simulink model "RB_KAIROS_BaseOnly"  (R2020b)
settings: Solver=ode4  StartTime=0.0  StopTime=t_end  FixedStep=Ts  RelTol=1e-3
values from neighbouring files (symbols this model uses):
  am = 0.3    [RB_KAIROS_ImpControl_OpSpace_BaseOnly.m]
  am_r = 0.3    [RB_KAIROS_ImpControl_OpSpace_BaseOnly.m]
  Jv = [1 0 0; 0 1 0; 0 0 0; 0 0 0; 0 0 0; 0 0 1;]    [RB_KAIROS_ImpControl_OpSpace_BaseOnly.m]
  Kc = diag(5*[1000,1000,0,0,0,1000])    [RB_KAIROS_ImpControl_OpSpace_BaseOnly.m]
  model_sample_time = 0.001    [RB_KAIROS_ImpControl_OpSpace_BaseOnly.m]
  q_dot_0 = zeros(10,1)    [RB_KAIROS_ImpControl_OpSpace_BaseOnly.m]
  T_i = T_W_V    [RB_KAIROS_ImpControl_OpSpace_BaseOnly.m]
  tau_ext = [0 0 0]    [RB_KAIROS_ImpControl_OpSpace_BaseOnly.m]
  v_SMU = 10    [RB_KAIROS_ImpControl_OpSpace_BaseOnly.m]
  vm = 0.6    [RB_KAIROS_ImpControl_OpSpace_BaseOnly.m]
  vm_r = 0.6    [RB_KAIROS_ImpControl_OpSpace_BaseOnly.m]
undefined symbols (not defined in the file or in its folder): DiscIntNeverNeededParam, magnitude, q_0, T_f
libraries: simulink x4, utils x4, transformations_lib x1
(part 14 of 16)

== matlab function RB_KAIROS_BaseOnly/CONTROLLER /Kinematics and Dynamics/Kinematics - error representation/MATLAB Function2 ==
  data: R_D_W_aug input; vt output; x_dot_d input; x_ddot_d input; vt_dot output; x_err input; x_dot_err input
function [vt, vt_dot] = compute_vt(R_D_W_aug, x_dot_d, x_ddot_d, x_err, x_dot_err)
% This function is used to compute the vectors vt and vt_dot defined in Ott book in order
% to convert the equation of motion to an equivalent representation using
% error on the task variables

% INPUTS:
% - R_W_D_aug is an extension of the ROTATION MATRIX from world frame to 
%   desired frame: [R_W_D 0; 0 R_W_D], it is a 6x6 matrix
% - omega_d, p_dot_d, p_err, eps_err, omega_err are all quantities defined in
%   the world frame (or space frame) W.
S_omega_d = calc_skewsymm(x_dot_d(4:6));
S_alfa_d = calc_skewsymm(x_ddot_d(4:6));

a = [x_dot_d(1:3) + S_omega_d*(x_err(1:3));
                x_dot_d(4:6)];

vt = R_D_W_aug*a;

vt_dot = R_D_W_aug*(-augment_matrix(S_omega_d)*a + [x_ddot_d(1:3) + S_alfa_d*x_err(1:3) + S_omega_d*x_dot_err(1:3);
                                                                  x_ddot_d(4:6)]);

end 


function S = calc_skewsymm(v)

S = [0 -v(3) v(2);
    v(3) 0 -v(1);
    -v(2) v(1) 0];
end

function M_aug = augment_matrix(M)

M_aug = [M, zeros(3,3);
             zeros(3,3), M];
end

== matlab function RB_KAIROS_BaseOnly/CONTROLLER /Kinematics and Dynamics/Kinematics - error representation/MATLAB Function3 ==
  data: R_D_W_aug input; J_x output; J_b input
function J_x   =compute_J_x(R_D_W_aug, J_b)
% This function is used to compute the matrix J_x defined in Ott book in order
% to convert the equation of motion to an equivalent representation using
% error on the task variables

% INPUTS:
% - R_W_D_aug is an extension of the ROTATION MATRIX from world frame to 
%   desired frame: [R_W_D 0; 0 R_W_D], it is a 6x6 matrix
% - J_b is the body Jacobian of the robot 

J_x = R_D_W_aug*J_b;

== matlab function RB_KAIROS_BaseOnly/CONTROLLER /Primary task - Controller/MATLAB Function ==
  data: Kc input; Dc output; Lambda input
function Dc = compute_damping(Kc,Lambda)
%  COMPUTE_DAMPING Computes damping matrix to enforce desired second order
%  system behaviour.
%
%   Dc = COMPUTE_DAMPING(Kc,Lambda) computes the damping depending on 
%        stiffness matrix Kc (which has to be constant for stability) and
%        inertia matrix Lambda (which is time varying since no inertia 
%        shaping is applied).
%   
%   Reference: Cartesian Impedance Control of Redundant and Flexible-Joint
%              Robots, C. Ott 2005, page 36-37.
%   See also EIG

zeta = 1;

Lambda_3 = Lambda([1:2,6],[1:2,6]);
Kc_3 = Kc([1:2,6],[1:2,6])

A = real(sqrtm(Lambda_3));
Kc_1 = real(sqrtm(Kc_3));

D0 = zeta*eye(3,3);

Dc_3 = A*D0*Kc_1 + Kc_1*D0*A;

Dc = zeros(6,6);

Dc([1:2,6],[1:2,6]) = Dc_3

% DAMPING MATRIX (varying)
%Generalized eigenvalue decomposition for the pair (Kc,Lambda)
% Lambda_3 = Lambda([1:2,6],[1:2,6]);
% Kc_3 = Kc([1:2,6],[1:2,6]);
% [eigvecs,eigvals] =  eig(Kc_3, Lambda_3);
% eigvals = real(eigvals);
% eigvecs = real(eigvecs);
% %sorting eigs by magnitude
% % [eigvals,sidx] = sort(diag(eigvals),'descend');
% 
% %Finding matrices that satisfy K = Q'K0Q and Lambda = Q'*Q
% K0_3 = sqrt(eigvals);
% % V = eigvecs(:,sidx);
% Q_T = Lambda_3*eigvecs;
% Q = Q_T';
% 
% %Damping matrix computation
% zeta = 1*ones(3,1); %Imposing an overdamped behaviour
% D0_3 = diag(zeta).*K0_3;
% Dc_3 = 2*Q_T*D0_3*Q;
% 
% Dc = eye(6);
% Dc([1:2,6],[1:2,6]) = Dc_3

%OLD implementation where stiffness and damping were retrieven from
%configuration parameters
% function [Kc,Dc] = compute_stiffness_damping(J_T, J_i, J_d)
% 
% Kq_veh = [2850*ones(2,1); 750]; 
% Dq_veh = [2000;2000;800];
% 
% Kq = diag([Kq_veh]);
% Dq = diag([Dq_veh]);
% 
% Dc = J_i'*Dq*J_i;
% Kc = J_i'*(Kq-J_T*Dc*J_d)*J_i;
% end

== matlab function RB_KAIROS_BaseOnly/EE to task space quaternion quantities/Augment matrix ==
  data: R_W_D input; R_D_W_aug output
function R_D_W_aug = augment_matrix(R_W_D)

R_D_W_aug = [R_W_D', zeros(3,3);
             zeros(3,3), R_W_D'];

== matlab function RB_KAIROS_BaseOnly/Trajectory Generator/move2pose/Cartesian_ipol2/rotation/Embedded MATLAB Function1 ==
  data: t input; qd output; s0 input; v0 input; sf input; vm input; am input; dqd output; ddqd output; ipol_finished output; T_scale input; interpoly input
function [qd,dqd,ddqd, ipol_finished] = calc_qd(t,s0,v0,sf,vm,am,T_scale,interpoly)
% This function calculates a one dimensional movement with a trapezodial 
% signal for velocity over time. Additionally it is able to adapt to shifts
% in the maximum allowed velocity.
%
% Inputs:
% t         current runtime
% s0        start value for motion in position
% v0        start value for motion in velocity
% sf        final value for motion in position
% vm        maximum allowed velocity
% am        maximum allowed acceleration
% T_scale   Scaling factor for duration of adaption
% interpoly Which interpolation to use
%
% Outputs:
% qd        disered position at current time
% dqd       disered velocity at current time
% ddqd      disered acceleration at current time
% ipol_finished 
%           motion is finished

%% Initialize persistent variables for adaption motion
persistent vm1 adpt ti qi qf T t_shift
if isempty(vm1)
    vm1 = vm;       %remembers the max velocity from last run
end
if isempty(adpt)
    adpt = false;   %stores if an adaption motion is activated
end
if isempty(ti)
    ti = 0;         %Initial time step for adaption motion
end
if isempty(qi)
    qi = zeros(3,1);%Initial values (pos,vel,acc) for adaption motion
end
if isempty(qf)
    qf = zeros(3,1);%Final values (pos,vel,acc) for adaption motion
end
if isempty(T)
    T = 0;          %Duration of adaption motion; tf = ti+T
end
if isempty(t_shift)
    t_shift = 0;    %Time distance with which the current reference motion is shifted
end

% needed to delay tanhlog with one timestep
tanhlog_delay = 0;

%% This If runs only for one timestep!!!
% If current max velocity is unequal to old one 
% Not directly at the beginning
% Dont start new while a adaption is still running, to prevent reset of
%   initial values
if abs(vm-vm1)>1e-3 && t>0.001 && adpt==false                       
    adpt = true;          % Activate adaption
    ti = t;               % Set initial timestep to current step
    tanhlog_delay = 1;    % Activate the delay for tanhlog

    %%% inital set of position, velo, acceleration for adaption motion 
    % is the same as the old mogen would do (t_shift is not updated at
    % this time!)
    [qi, ~] = interpolator(ti+t_shift, compute_traj_parameters(s0, v0, sf, vm1, am));

    %%% computes the time shift for shifting the new motion to the end
    % point of the old motion. So at which time the new motion has
    % the same qd? Then calculate the time distance to the inital
    % time of the change in velocities
    % t_shift < 0 if new motion is faster (vm>vm1)
    % t_shift > 0 if new motion is slower (vm<vm1)
    % interpolator_1 is the inverse function of interpolator!
    t_shift = interpolator_1(qi(1), compute_traj_parameters(s0, v0, sf, vm, am)) - ti ;

    %%% Additional shift for adaption motion = Duration of adaption motion
    T_standard = abs(vm1-vm)/am;
    switch interpoly
        case 0
            T = 0;
            adpt = false;       %no adatption  
        case 1
            T = T_standard*2.2;    %tanhlog
        case 2
            T = (pi*abs(vm1-vm))/(2*am);  %Cosine version
        case 3
            T = T_standard;        %poly3
        case 4
            T = 1.5*(abs(vm1-vm)/am); %poly4
        case 5
            T = T_standard*1.5;        %poly5 
        case 7
            T = T_standard*1.75;        %poly7 
        otherwise
            T = T_standard;        %rest
    end

    % Scale Duration if needed
    T = T*T_scale;

    %%% The additional shift for adaption motion is dependent on the
    % difference in the velocities. See report for details.
    t_shift  = t_shift+(T/2)*((vm1/vm)-1);

    %%% Calculate final values for adaption motion. Which are reached
    % at inital time plus duration of adaption and new time shift
    [qf, ~] = interpolator(ti+t_shift+T, compute_traj_parameters(s0, v0, sf, vm, am));

end

%% Here the actual motion is calculated
% Interpolates the values of pos,vel,acc (qv) with parameters and current time t    
[qdv, ipol_finished] = interpolator(t+t_shift, compute_traj_parameters(s0, v0, sf, vm, am));  

%% If adaption motion needed
if adpt == true 

    %%% calculate the adaption moition, which takes time from ti to
    % ti+T. t is the current runtime, _i initial values, _f final
    % values, _m maximum values

    switch interpoly
        case 0
            adpt=false;                             %no adatption  
        case 1
            if tanhlog_delay == 1
                qdv = qi;  
                tanhlog_delay = 0;
            else
                qdv = tanhlog(t,ti,T,qi,qf,vm,am);      %tanhlog
            end
        case 2
            qdv = cosine(t,ti,T,qi,qf,vm,am);       %Cosine version
        case 3
            qdv = poly3(t,ti,T,qi,qf,vm,am);        %poly3
        case 4
            qdv = poly4(t,ti,T,qi,qf,vm,am);        %poly4
        case 5
            qdv = poly5(t,ti,T,qi,qf,vm,am);        %poly5 
        case 6
            qdv = poly6(t,ti,T,qi,qf,vm,am);        %poly6 
        case 7
            qdv = poly7(t,ti,T,qi,qf,vm,am);        %poly7 
        case 8
            qdv = poly4_mean(t,ti,T,qi,qf,vm,am);   %poly4_mean 
        case 9
            qdv = poly5_2mean(t,ti,T,qi,qf,vm,am);  %poly5_2mean 
        case 10
            qdv = tanhmean(t,ti,T,qi,qf,vm,am);     %tanhmean 
        otherwise
            error('Unknown adaption motion');       %rest
    end

    % If time is equal than the finish time => adaption motion is complete
    % But it is aborted one timestep earlier, since the finish timestep
    % is already computed correctly by the standard interpolator.
    if t >= (ti+T-0.001)
        adpt = false;     % If adaption finished => reset
    end
end

%% Set output
if sf == s0          % No motion needed if start = end 
    qd = s0;         % => set initial values
    dqd = v0;
    ddqd = 0;  
else     
    qd = qdv(1);     % set output
    dqd = qdv(2);
    ddqd = qdv(3);        
end

vm1 = vm;  %remember current max velocity

end

function [qv] = poly3(t,ti,T,qvi,qvf,dqm,ddqm)
%POLY3 computes a polynomial trajectory of degree 3 between initial (_i) 
%values and final (_f) values of position q, velocity dq and accelerataion
%ddq. Taken from Melchiorri presentation page 19

qi = qvi(1);      %split input vectors in pos,vel,acc
dqi = qvi(2);
ddqi = qvi(3);
qf = qvf(1);
dqf = qvf(2);
ddqf = qvf(3);
      
% current duration of motion dt
dt = t-ti;                      

% compute coefficients
a0 = qi;
a1 = dqi;
a2 = (-3*(qi-qf)-(2*dqi+dqf)*T)/(T^2);
a3 = (2*(qi-qf)+(dqi+dqf)*T)/(T^3);

% compute pos,vel,acc desired (_d)
qd = a0+a1*dt+a2*dt^2+a3*dt^3;
dqd = a1+2*a2*dt+3*a3*dt^2;
ddqd = 2*a2+6*a3*dt;

qv = [qd;dqd;ddqd]; %Send values back

end

function [qv] = poly4(t,ti,T,qvi,qvf,dqm,ddqm)
%POLY4 computes a polynomial trajectory of degree 4 between initial (_i) 
%values and final (_f) values of position q, velocity dq and accelerataion
%ddq. inspired by old function in here

qi = qvi(1);      %split input vectors in pos,vel,acc
dqi = qvi(2);
ddqi = qvi(3);
qf = qvf(1);
dqf = qvf(2);
ddqf = qvf(3);
      
% current duration of motion dt
dt = t-ti;                      

% a2 = 0;
% a3 = -4/9*ddqm^2/(dqi-dqm);
% a4 = -4/27*ddqm^3/(dqi-dqm)^2;
a2 = 0;
a3 = -4/9*ddqm^2/abs(dqi-dqf);
a4 = 4/27*ddqm^3/abs(dqi-dqf)^2;

a0 = qi;
a1 = dqi;
% a2 = 0.5*ddqi;
% a3 = (4*(qf-qi)-(dqf+3*dqi)*T-ddqi*(T^2))/(T^3);
% a4 = (3*(qi-qf)+(dqf+2*dqi)*T+0.5*ddqi*(T^2))/(T^4);

% compute pos,vel,acc desired (_d)
qd = (a4*dt^4+a3*dt^3+a2*dt^2+a1*dt+a0);
dqd = 4*a4*dt^3+3*a3*dt^2+2*a2*dt+a1;
ddqd = 12*a4*dt^2+6*a3*dt+2*a2;

qv = [qd;dqd;ddqd]; %Send values back

end

function [qv] = poly4_mean(t,ti,T,qvi,qvf,dqm,ddqm)
%POLY4 computes a polynomial trajectory of degree 4 between initial (_i) 
%values and final (_f) values of position q, velocity dq and accelerataion
%ddq with mean velocity at T/2. self made

qi = qvi(1);      %split input vectors in pos,vel,acc
dqi = qvi(2);
ddqi = qvi(3);
qf = qvf(1);
dqf = qvf(2);
ddqf = qvf(3);
      
% current duration of motion dt
dt = t-ti;                     

b = [qi dqi qf dqf 0.5*(dqi+dqf)]';

M_inv = [...
       1,     0,      0,          0,           0;
       0,     1,      0,          0,           0;
   6/T^2,  -2/T, -6/T^2,    5/(4*T),    27/(4*T);
 -16/T^3, 1/T^2, 16/T^3, -7/(2*T^2), -27/(2*T^2);
   9/T^4,     0, -9/T^4,  9/(4*T^3),  27/(4*T^3)];

a = M_inv * b;

% compute pos,vel,acc desired (_d)

qd = a(1)+a(2)*dt+a(3)*dt^2+a(4)*dt^3+a(5)*dt^4;
dqd = a(2)+2*a(3)*dt+3*a(4)*dt^2+4*a(5)*dt^3;
ddqd = 2*a(3)+6*a(4)*dt+12*a(5)*dt^2;

qv = [qd;dqd;ddqd]; %Send values back

end

function [qv] = poly5(t,ti,T,qvi,qvf,dqm,ddqm)
%POLY5 computes a polynomial trajectory of degree 5 between initial (_i) 
%values and final (_f) values of position q, velocity dq and accelerataion
%ddq. Taken from Melchiorri presentation page 25

qi = qvi(1);      %split input vectors in pos,vel,acc
dqi = qvi(2);
ddqi = qvi(3);
qf = qvf(1);
dqf = qvf(2);
ddqf = qvf(3);
      
% current duration of motion dt
dt = t-ti;                      

% compute coefficients
a0 = qi;
a1 = dqi;
a2 = 0.5*ddqi;
a3 = (20*(qf-qi)-(8*dqf+12*dqi)*T-(3*ddqf-ddqi)*T^2)/(2*T^3);
a4 = (30*(qi-qf)+(14*dqf+16*dqi)*T+(3*ddqf-2*ddqi)*T^2)/(2*T^4);
a5 = (12*(qf-qi)-6*(dqf+dqi)*T-(ddqf-ddqi)*T^2)/(2*T^5);

% compute pos,vel,acc desired (_d)
qd = a0+a1*dt+a2*dt^2+a3*dt^3+a4*dt^4+a5*dt^5;
dqd = a1+2*a2*dt+3*a3*dt^2+4*a4*dt^3+5*a5*dt^4;
ddqd = 2*a2+6*a3*dt+12*a4*dt^2+20*a5*dt^3;

qv = [qd;dqd;ddqd]; %Send values back

end

function [qv] = poly5_2mean(t,ti,T,qvi,qvf,dqm,ddqm)
%POLY5 computes a polynomial trajectory of degree 5 between initial (_i) 
%values and final (_f) values of position q, velocity dq and accelerataion
%ddq with 2*mean steps at T/3 and 2T/3. self made

qi = qvi(1);      %split input vectors in pos,vel,acc
dqi = qvi(2);
ddqi = qvi(3);
qf = qvf(1);
dqf = qvf(2);
ddqf = qvf(3);
      
% current duration of motion dt
dt = t-ti;                      

% compute coefficients
b = [qi dqi qf dqf 0.5*(dqi+dqf)+(1/6)*(dqi-dqf) 0.5*(dqi+dqf)+(1/6)*(dqi-dqf)]';

M_inv = [...
        1,          0,        0,           0,            0,           0;
        0,          1,        0,           0,            0,           0;
  -30/T^2,  -13/(2*T),   30/T^2,   -13/(4*T),    -27/(4*T),   -27/(2*T);
  110/T^3, 67/(4*T^2), -110/T^3,  49/(4*T^2),  135/(4*T^2), 189/(4*T^2);
 -135/T^4,    -18/T^3,  135/T^4, -63/(4*T^3), -189/(4*T^3),     -54/T^3;
   54/T^5, 27/(4*T^4),  -54/T^5,  27/(4*T^4),   81/(4*T^4),  81/(4*T^4)];

a = M_inv * b;

% compute pos,vel,acc desired (_d)

qd = a(1)+a(2)*dt+a(3)*dt^2+a(4)*dt^3+a(5)*dt^4+a(6)*dt^5;
dqd = a(2)+2*a(3)*dt+3*a(4)*dt^2+4*a(5)*dt^3+5*a(6)*dt^4;
ddqd = 2*a(3)+6*a(4)*dt+12*a(5)*dt^2+20*a(6)*dt^3;

qv = [qd;dqd;ddqd]; %Send values back

end

function [qv] = poly6(t,ti,T,qvi,qvf,dqm,ddqm)
%POLY6 computes a polynomial trajectory of degree 6 between initial (_i) 
%values and final (_f) values of position q, velocity dq and accelerataion
%ddq with mean velocity at T/3. self made

qi = qvi(1);      %split input vectors in pos,vel,acc
dqi = qvi(2);
ddqi = qvi(3);
qf = qvf(1);
dqf = qvf(2);
ddqf = qvf(3);

% current duration of motion dt
dt = t-ti;                      

% compute coefficients
b = [qi dqi 0.5*ddqi qf dqf ddqf 0.5*(dqi+dqf)]';

M_inv = [...
       1,      0,      0,       0,           0,          0,            0;
       0,      1,      0,       0,           0,          0,            0;
       0,      0,      1,       0,           0,          0,            0;
  20/T^3, -6/T^2,   -4/T, -20/T^3,  23/(4*T^2),   -1/(2*T),   81/(4*T^2);
 -75/T^4,  8/T^3,  6/T^2,  75/T^4, -89/(4*T^3),      2/T^2, -243/(4*T^3);
  84/T^5, -3/T^4, -4/T^3, -84/T^5, 105/(4*T^4), -5/(2*T^3),  243/(4*T^4);
 -30/T^6,      0,  1/T^4,  30/T^6, -39/(4*T^5),      1/T^4,  -81/(4*T^5)];

a = M_inv * b;

% compute pos,vel,acc desired (_d)

qd = a(1)+a(2)*dt+a(3)*dt^2+a(4)*dt^3+a(5)*dt^4+a(6)*dt^5+a(7)*dt^6;
dqd = a(2)+2*a(3)*dt+3*a(4)*dt^2+4*a(5)*dt^3+5*a(6)*dt^4+6*a(7)*dt^5;
ddqd = 2*a(3)+6*a(4)*dt+12*a(5)*dt^2+20*a(6)*dt^3+30*a(7)*dt^4;

qv = [qd;dqd;ddqd]; %Send values back

end

function [qv] = poly7(t,ti,T,qvi,qvf,dqm,ddqm)
%POLY7 computes a polynomial trajectory of degree 7 between initial (_i) 
%values and final (_f) values of position q, velocity dq, accelerataion
%ddq and jerk dddq. self made

qi = qvi(1);      %split input vectors in pos,vel,acc
dqi = qvi(2);
ddqi = qvi(3);
dddqi = 0;
qf = qvf(1);
dqf = qvf(2);
ddqf = qvf(3);
dddqf = 0;

% current duration of motion dt
dt = t-ti;                      

% compute coefficients
 
a = [...
                                                                                                                                                                            conj(qi)
                                                                                                                                                                           conj(dqi)
                                                                                                                                                                        conj(ddqi)/2
                                                                                                                                                                       conj(dddqi)/6
           (5*conj(ddqf))/(2*T^2) - (2*conj(dddqi))/(3*T) - conj(dddqf)/(6*T) - (5*conj(ddqi))/T^2 - (15*conj(dqf))/T^3 - (20*conj(dqi))/T^3 + (35*conj(qf))/T^4 - (35*conj(qi))/T^4
                  conj(dddqf)/(2*T^2) + conj(dddqi)/T^2 - (7*conj(ddqf))/T^3 + (10*conj(ddqi))/T^3 + (39*conj(dqf))/T^4 + (45*conj(dqi))/T^4 - (84*conj(qf))/T^5 + (84*conj(qi))/T^5
 (13*conj(ddqf))/(2*T^4) - (2*conj(dddqi))/(3*T^3) - conj(dddqf)/(2*T^3) - (15*conj(ddqi))/(2*T^4) - (34*conj(dqf))/T^5 - (36*conj(dqi))/T^5 + (70*conj(qf))/T^6 - (70*conj(qi))/T^6
               conj(dddqf)/(6*T^4) + conj(dddqi)/(6*T^4) - (2*conj(ddqf))/T^5 + (2*conj(ddqi))/T^5 + (10*conj(dqf))/T^6 + (10*conj(dqi))/T^6 - (20*conj(qf))/T^7 + (20*conj(qi))/T^7];
 


% compute pos,vel,acc desired (_d)

qd = a(1)+a(2)*dt+a(3)*dt^2+a(4)*dt^3+a(5)*dt^4+a(6)*dt^5+a(7)*dt^6+a(8)*dt^7;
dqd = a(2)+2*a(3)*dt+3*a(4)*dt^2+4*a(5)*dt^3+5*a(6)*dt^4+6*a(7)*dt^5+7*a(8)*dt^6;
ddqd = 2*a(3)+6*a(4)*dt+12*a(5)*dt^2+20*a(6)*dt^3+30*a(7)*dt^4+42*a(8)*dt^5;

qv = [qd;dqd;ddqd]; %Send values back

end

function [qv] = cosine(t,ti,T,qvi,qvf,dqm,ddqm)
%COSINE computes a cosine trajectory between initial (_i) 
%values and final (_f) values of position q, velocity dq and accelerataion
%ddq with respect to the maximum values (_m). t is the current runtime

qi = qvi(1);      %split input vectors in pos,vel,acc
dqi = qvi(2);
ddqi = qvi(3);
qf = qvf(1);
dqf = qvf(2);
ddqf = qvf(3);
      
% often needed values

%T = (pi*abs(dqf-dqi))/(2*ddqm); % total duration of motion T (with am)
%T = abs((2*(qf-qi))/(dqi-dqf));
dt = t-ti;                      % current duration of motion dt

%cm = (T/(2*pi))*(dqm-(1/T)*(qf-qi));
c = qi-0.5*(dqi+dqf)*ti;
%cn = qf-0.5*(dqi+dqf)*(ti+T);
%c = cn + 0.5*(1+cos((pi/T)*dt))*(ca-cn);


% if t<(ti+(T/2))
%     c = qi - 0.5*(dqi+dqf)*ti;
% else
%     c = qf - 0.5*(((dqi+dqf)/2)+dqf)*tf;
% end

%c = (qi+qf)/2 - 0.5*(dqi+dqf)*(ti+(T/2)) - 0.5*(dqi-dqf)*(T/pi);
% compute pos,vel,acc desired (_d)
%qd = qi + (1/T)*(qf-qi)*dt + cm*sin(((2*pi)/T)*dt);
qd = 0.5*(dqi+dqf)*t + 0.5*(T/pi)*(dqi-dqf)*sin((pi/T)*dt) + c;
dqd = 0.5*(dqi+dqf) + 0.5*(dqi-dqf)*cos((pi/T)*dt);
ddqd = -0.5*(pi/T)*(dqi-dqf)*sin((pi/T)*dt);

qv = [qd;dqd;ddqd]; %Send values back

end

function [qv] = tanhmean(t,ti,T,qvi,qvf,dqm,ddqm)
%TANHMEAN computes a tanh trajectory between initial (_i) 
%values and final (_f) values of position q, velocity dq and accelerataion
%ddq with respect to the maximum values (_m). t is the current runtime
%selfmade

qi = qvi(1);      %split input vectors in pos,vel,acc
dqi = qvi(2);
ddqi = qvi(3);
qf = qvf(1);
dqf = qvf(2);
ddqf = qvf(3);
      
% current duration of motion dt
dt = t-ti;                      
t_norm = dt/T;
theta = 4;

qd = 0.5*(1/theta)*(dqf-dqi)*log(cosh(theta*(t_norm-0.5))) ...
     + 0.5*(dqi+dqf)*t_norm ...
     + qf - 0.5*(1/theta)*(dqf-dqi)*log(cosh(0.5*theta));
     %+ qi - 0.5*(1/theta)*(dqf-dqi)*log(cosh(-0.5*theta));
dqd = 0.5*(dqi+dqf) + 0.5*(dqf-dqi)*tanh(theta*(t_norm-0.5));
ddqd = 0.5*theta*(dqf-dqi)*sech(t_norm-0.5)^2;

qv = [qd;dqd;ddqd]; %Send values back

end

function [qv] = tanhlog(t,ti,T,qvi,qvf,dqm,ddqm)
%TANHLOG computes a tanh-log trajectory between initial (_i) 
%values and final (_f) values of position q, velocity dq and accelerataion
%ddq with respect to the maximum values (_m). t is the current runtime
%taken from Internet

qi = qvi(1);      %split input vectors in pos,vel,acc
dqi = qvi(2);
ddqi = qvi(3);
qf = qvf(1);
dqf = qvf(2);
ddqf = qvf(3);
      
% current duration of motion dt
dt = t-ti;  

a = dqi;
b = qi;      
c = dqf;
d = qf-dqf*T;
k = d-b;

x = (a*dt+b-c*dt-d+k)/(2*k);
w = (tanh(((log(1-x))^2-(log(x))^2)/3)+1)/2;
p = tanh((log(2-x)-log(x))*(1-(1/sqrt(2))*(log(2-x)+log(x))))+2*x-1;
q = tanh((log(x+1)-log(1-x))*(1-(1/sqrt(2))*(log(1-x)+log(x+1))));
s = p*(1-w)+q*w;

qd = k*s+c*dt+d-k;

dqd = dqf + (qi - qf + T*dqf)*((tanh(log((dqf*dt - dqi*dt)/(2*qi - 2*qf + 2*T*dqf))^2/3 - log(1 - (dqf*dt - dqi*dt)/(2*qi - 2*qf + 2*T*dqf))^2/3)/2 + 1/2)*((((2^(1/2)*(log(2 - (dqf*dt - dqi*dt)/(2*qi - 2*qf + 2*T*dqf)) + log((dqf*dt - dqi*dt)/(2*qi - 2*qf + 2*T*dqf))))/2 - 1)*((dqf - dqi)/(dqf*dt - dqi*dt) - (dqf - dqi)/(((dqf*dt - dqi*dt)/(2*qi - 2*qf + 2*T*dqf) - 2)*(2*qi - 2*qf + 2*T*dqf))) - (2^(1/2)*(log(2 - (dqf*dt - dqi*dt)/(2*qi - 2*qf + 2*T*dqf)) - log((dqf*dt - dqi*dt)/(2*qi - 2*qf + 2*T*dqf)))*((dqf - dqi)/(dqf*dt - dqi*dt) + (dqf - dqi)/(((dqf*dt - dqi*dt)/(2*qi - 2*qf + 2*T*dqf) - 2)*(2*qi - 2*qf + 2*T*dqf))))/2)*(tanh((log(2 - (dqf*dt - dqi*dt)/(2*qi - 2*qf + 2*T*dqf)) - log((dqf*dt - dqi*dt)/(2*qi - 2*qf + 2*T*dqf)))*((2^(1/2)*(log(2 - (dqf*dt - dqi*dt)/(2*qi - 2*qf + 2*T*dqf)) + log((dqf*dt - dqi*dt)/(2*qi - 2*qf + 2*T*dqf))))/2 - 1))^2 - 1) - (2*(dqf - dqi))/(2*qi - 2*qf + 2*T*dqf)) - (tanh(((2^(1/2)*(log((dqf*dt - dqi*dt)/(2*qi - 2*qf + 2*T*dqf) + 1) + log(1 - (dqf*dt - dqi*dt)/(2*qi - 2*qf + 2*T*dqf))))/2 - 1)*(log((dqf*dt - dqi*dt)/(2*qi - 2*qf + 2*T*dqf) + 1) - log(1 - (dqf*dt - dqi*dt)/(2*qi - 2*qf + 2*T*dqf))))^2 - 1)*(tanh(log((dqf*dt - dqi*dt)/(2*qi - 2*qf + 2*T*dqf))^2/3 - log(1 - (dqf*dt - dqi*dt)/(2*qi - 2*qf + 2*T*dqf))^2/3)/2 - 1/2)*(((2^(1/2)*(log((dqf*dt - dqi*dt)/(2*qi - 2*qf + 2*T*dqf) + 1) + log(1 - (dqf*dt - dqi*dt)/(2*qi - 2*qf + 2*T*dqf))))/2 - 1)*((dqf - dqi)/(((dqf*dt - dqi*dt)/(2*qi - 2*qf + 2*T*dqf) - 1)*(2*qi - 2*qf + 2*T*dqf)) - (dqf - dqi)/(((dqf*dt - dqi*dt)/(2*qi - 2*qf + 2*T*dqf) + 1)*(2*qi - 2*qf + 2*T*dqf))) - (2^(1/2)*(log((dqf*dt - dqi*dt)/(2*qi - 2*qf + 2*T*dqf) + 1) - log(1 - (dqf*dt - dqi*dt)/(2*qi - 2*qf + 2*T*dqf)))*((dqf - dqi)/(((dqf*dt - dqi*dt)/(2*qi - 2*qf + 2*T*dqf) - 1)*(2*qi - 2*qf + 2*T*dqf)) + (dqf - dqi)/(((dqf*dt - dqi*dt)/(2*qi - 2*qf + 2*T*dqf) + 1)*(2*qi - 2*qf + 2*T*dqf))))/2) + (tanh(((2^(1/2)*(log((dqf*dt - dqi*dt)/(2*qi - 2*qf + 2*T*dqf) + 1) + log(1 - (dqf*dt - dqi*dt)/(2*qi - 2*qf + 2*T*dqf))))/2 - 1)*(log((dqf*dt - dqi*dt)/(2*qi - 2*qf + 2*T*dqf) + 1) - log(1 - (dqf*dt - dqi*dt)/(2*qi - 2*qf + 2*T*dqf))))*((2*log((dqf*dt - dqi*dt)/(2*qi - 2*qf + 2*T*dqf))*(dqf - dqi))/(3*(dqf*dt - dqi*dt)) - (2*log(1 - (dqf*dt - dqi*dt)/(2*qi - 2*qf + 2*T*dqf))*(dqf - dqi))/(3*((dqf*dt - dqi*dt)/(2*qi - 2*qf + 2*T*dqf) - 1)*(2*qi - 2*qf + 2*T*dqf)))*(tanh(log((dqf*dt - dqi*dt)/(2*qi - 2*qf + 2*T*dqf))^2/3 - log(1 - (dqf*dt - dqi*dt)/(2*qi - 2*qf + 2*T*dqf))^2/3)^2 - 1))/2 - (((2*log((dqf*dt - dqi*dt)/(2*qi - 2*qf + 2*T*dqf))*(dqf - dqi))/(3*(dqf*dt - dqi*dt)) - (2*log(1 - (dqf*dt - dqi*dt)/(2*qi - 2*qf + 2*T*dqf))*(dqf - dqi))/(3*((dqf*dt - dqi*dt)/(2*qi - 2*qf + 2*T*dqf) - 1)*(2*qi - 2*qf + 2*T*dqf)))*(tanh(log((dqf*dt - dqi*dt)/(2*qi - 2*qf + 2*T*dqf))^2/3 - log(1 - (dqf*dt - dqi*dt)/(2*qi - 2*qf + 2*T*dqf))^2/3)^2 - 1)*(tanh((log(2 - (dqf*dt - dqi*dt)/(2*qi - 2*qf + 2*T*dqf)) - log((dqf*dt - dqi*dt)/(2*qi - 2*qf + 2*T*dqf)))*((2^(1/2)*(log(2 - (dqf*dt - dqi*dt)/(2*qi - 2*qf + 2*T*dqf)) + log((dqf*dt - dqi*dt)/(2*qi - 2*qf + 2*T*dqf))))/2 - 1)) - (2*(dqf*dt - dqi*dt))/(2*qi - 2*qf + 2*T*dqf) + 1))/2);

ddqd = -(qi - qf + T*dqf)*(((tanh(log((dqf*dt - dqi*dt)/(2*qi - 2*qf + 2*T*dqf))^2/3 - log(1 - (dqf*dt - dqi*dt)/(2*qi - 2*qf + 2*T*dqf))^2/3)^2 - 1)*(tanh((log(2 - (dqf*dt - dqi*dt)/(2*qi - 2*qf + 2*T*dqf)) - log((dqf*dt - dqi*dt)/(2*qi - 2*qf + 2*T*dqf)))*((2^(1/2)*(log(2 - (dqf*dt - dqi*dt)/(2*qi - 2*qf + 2*T*dqf)) + log((dqf*dt - dqi*dt)/(2*qi - 2*qf + 2*T*dqf))))/2 - 1)) - (2*(dqf*dt - dqi*dt))/(2*qi - 2*qf + 2*T*dqf) + 1)*((2*(dqf - dqi)^2)/(3*(dqf*dt - dqi*dt)^2) - (2*(dqf - dqi)^2)/(3*((dqf*dt - dqi*dt)/(2*qi - 2*qf + 2*T*dqf) - 1)^2*(2*qi - 2*qf + 2*T*dqf)^2) - (2*log((dqf*dt - dqi*dt)/(2*qi - 2*qf + 2*T*dqf))*(dqf - dqi)^2)/(3*(dqf*dt - dqi*dt)^2) + (2*log(1 - (dqf*dt - dqi*dt)/(2*qi - 2*qf + 2*T*dqf))*(dqf - dqi)^2)/(3*((dqf*dt - dqi*dt)/(2*qi - 2*qf + 2*T*dqf) - 1)^2*(2*qi - 2*qf + 2*T*dqf)^2)))/2 - (tanh(((2^(1/2)*(log((dqf*dt - dqi*dt)/(2*qi - 2*qf + 2*T*dqf) + 1) + log(1 - (dqf*dt - dqi*dt)/(2*qi - 2*qf + 2*T*dqf))))/2 - 1)*(log((dqf*dt - dqi*dt)/(2*qi - 2*qf + 2*T*dqf) + 1) - log(1 - (dqf*dt - dqi*dt)/(2*qi - 2*qf + 2*T*dqf))))*(tanh(log((dqf*dt - dqi*dt)/(2*qi - 2*qf + 2*T*dqf))^2/3 - log(1 - (dqf*dt - dqi*dt)/(2*qi - 2*qf + 2*T*dqf))^2/3)^2 - 1)*((2*(dqf - dqi)^2)/(3*(dqf*dt - dqi*dt)^2) - (2*(dqf - dqi)^2)/(3*((dqf*dt - dqi*dt)/(2*qi - 2*qf + 2*T*dqf) - 1)^2*(2*qi - 2*qf + 2*T*dqf)^2) - (2*log((dqf*dt - dqi*dt)/(2*qi - 2*qf + 2*T*dqf))*(dqf - dqi)^2)/(3*(dqf*dt - dqi*dt)^2) + (2*log(1 - (dqf*dt - dqi*dt)/(2*qi - 2*qf + 2*T*dqf))*(dqf - dqi)^2)/(3*((dqf*dt - dqi*dt)/(2*qi - 2*qf + 2*T*dqf) - 1)^2*(2*qi - 2*qf + 2*T*dqf)^2)))/2 - (tanh(log((dqf*dt - dqi*dt)/(2*qi - 2*qf + 2*T*dqf))^2/3 - log(1 - (dqf*dt - dqi*dt)/(2*qi - 2*qf + 2*T*dqf))^2/3)/2 + 1/2)*((tanh((log(2 - (dqf*dt - dqi*dt)/(2*qi - 2*qf + 2*T*dqf)) - log((dqf*dt - dqi ...
    *dt)/(2*qi - 2*qf + 2*T*dqf)))*((2^(1/2)*(log(2 - (dqf*dt - dqi*dt)/(2*qi - 2*qf + 2*T*dqf)) + log((dqf*dt - dqi*dt)/(2*qi - 2*qf + 2*T*dqf))))/2 - 1))^2 - 1)*((2^(1/2)*(log(2 - (dqf*dt - dqi*dt)/(2*qi - 2*qf + 2*T*dqf)) - log((dqf*dt - dqi*dt)/(2*qi - 2*qf + 2*T*dqf)))*((dqf - dqi)^2/(dqf*dt - dqi*dt)^2 + (dqf - dqi)^2/(((dqf*dt - dqi*dt)/(2*qi - 2*qf + 2*T*dqf) - 2)^2*(2*qi - 2*qf + 2*T*dqf)^2)))/2 - ((dqf - dqi)^2/(dqf*dt - dqi*dt)^2 - (dqf - dqi)^2/(((dqf*dt - dqi*dt)/(2*qi - 2*qf + 2*T*dqf) - 2)^2*(2*qi - 2*qf + 2*T*dqf)^2))*((2^(1/2)*(log(2 - (dqf*dt - dqi*dt)/(2*qi - 2*qf + 2*T*dqf)) + log((dqf*dt - dqi*dt)/(2*qi - 2*qf + 2*T*dqf))))/2 - 1) + 2^(1/2)*((dqf - dqi)/(dqf*dt - dqi*dt) + (dqf - dqi)/(((dqf*dt - dqi*dt)/(2*qi - 2*qf + 2*T*dqf) - 2)*(2*qi - 2*qf + 2*T*dqf)))*((dqf - dqi)/(dqf*dt - dqi*dt) - (dqf - dqi)/(((dqf*dt - dqi*dt)/(2*qi - 2*qf + 2*T*dqf) - 2)*(2*qi - 2*qf + 2*T*dqf)))) + 2*tanh((log(2 - (dqf*dt - dqi*dt)/(2*qi - 2*qf + 2*T*dqf)) - log((dqf*dt - dqi*dt)/(2*qi - 2*qf + 2*T*dqf)))*((2^(1/2)*(log(2 - (dqf*dt - dqi*dt)/(2*qi - 2*qf + 2*T*dqf)) + log((dqf*dt - dqi*dt)/(2*qi - 2*qf + 2*T*dqf))))/2 - 1))*(((2^(1/2)*(log(2 - (dqf*dt - dqi*dt)/(2*qi - 2*qf + 2*T*dqf)) + log((dqf*dt - dqi*dt)/(2*qi - 2*qf + 2*T*dqf))))/2 - 1)*((dqf - dqi)/(dqf*dt - dqi*dt) - (dqf - dqi)/(((dqf*dt - dqi*dt)/(2*qi - 2*qf + 2*T*dqf) - 2)*(2*qi - 2*qf + 2*T*dqf))) - (2^(1/2)*(log(2 - (dqf*dt - dqi*dt)/(2*qi - 2*qf + 2*T*dqf)) - log((dqf*dt - dqi*dt)/(2*qi - 2*qf + 2*T*dqf)))*((dqf - dqi)/(dqf*dt - dqi*dt) + (dqf - dqi)/(((dqf*dt - dqi*dt)/(2*qi - 2*qf + 2*T*dqf) - 2)*(2*qi - 2*qf + 2*T*dqf))))/2)^2*(tanh((log(2 - (dqf*dt - dqi*dt)/(2*qi - 2*qf + 2*T*dqf)) - log((dqf*dt - dqi*dt)/(2*qi - 2*qf + 2*T*dqf)))*((2^(1/2)*(log(2 - (dqf*dt - dqi*dt)/(2*qi - 2*qf + 2*T*dqf)) + log((dqf*dt - dqi*dt)/(2*qi - 2*qf + 2*T*dqf))))/2 - 1))^2 - 1)) + ((2*log((dqf*dt - dqi*dt)/(2*qi - 2*qf + 2*T*dqf))*(dqf - dqi))/(3*(dqf*dt - dqi*dt)) - (2*log(1 - (dqf*dt - dqi*dt)/(2*qi - 2*qf + 2*T*dqf))*(dqf - dqi))/(3*((dqf*dt - dqi*dt)/(2*qi - 2*qf + 2*T*dqf) - 1)*(2*qi - 2*qf + 2*T*dqf)))*(tanh(log((dqf*dt - dqi*dt)/(2*qi - 2*qf + 2*T*dqf))^2/3 - log(1 - (dqf*dt - dqi*dt)/(2*qi - 2*qf + 2*T*dqf))^2/3)^2 - 1)*((((2^(1/2)*(log(2 - (dqf*dt - dqi*dt)/(2*qi - 2*qf + 2*T*dqf)) + log((dqf*dt - dqi*dt)/(2*qi - 2*qf + 2*T*dqf))))/2 - 1)*((dqf - dqi)/(dqf*dt - dqi*dt) - (dqf - dqi)/(((dqf*dt - dqi*dt)/(2*qi - 2*qf + 2*T*dqf) - 2)*(2*qi - 2*qf + 2*T*dqf))) - (2^(1/2)*(log(2 - (dqf*dt - dqi*dt)/(2*qi - 2*qf + 2*T*dqf)) - log((dqf*dt - dqi*dt)/(2*qi - 2*qf + 2*T*dqf)))*((dqf - dqi)/(dqf*dt - dqi*dt) + (dqf - dqi)/(((dqf*dt - dqi*dt)/(2*qi - 2*qf + 2*T*dqf) - 2)*(2*qi - 2*qf + 2*T*dqf))))/2)*(tanh((log(2 - (dqf*dt - dqi*dt)/(2*qi - 2*qf + 2*T*dqf)) - log((dqf*dt - dqi*dt)/(2*qi - 2*qf + 2*T*dqf)))*((2^(1/2)*(log(2 - (dqf*dt - dqi*dt)/(2*qi - 2*qf + 2*T*dqf)) + log((dqf*dt - dqi*dt)/(2*qi - 2*qf + 2*T*dqf))))/2 - 1))^2 - 1) - (2*(dqf - dqi))/(2*qi - 2*qf + 2*T*dqf)) + (tanh(((2^(1/2)*(log((dqf*dt - dqi*dt)/(2*qi - 2*qf + 2*T*dqf) + 1) + log(1 - (dqf*dt - dqi*dt)/(2*qi - 2*qf + 2*T*dqf))))/2 - 1)*(log((dqf*dt - dqi*dt)/(2*qi - 2*qf + 2*T*dqf) + 1) - log(1 - (dqf*dt - dqi*dt)/(2*qi - 2*qf + 2*T*dqf))))^2 - 1)*(tanh(log((dqf*dt - dqi*dt)/(2*qi - 2*qf + 2*T*dqf))^2/3 - log(1 - (dqf*dt - dqi*dt)/(2*qi - 2*qf + 2*T*dqf))^2/3)/2 - 1/2)*(2^(1/2)*((dqf - dqi)/(((dqf*dt - dqi*dt)/(2*qi - 2*qf + 2*T*dqf) - 1)*(2*qi - 2*qf + 2*T*dqf)) + (dqf - dqi)/(((dqf*dt - dqi*dt)/(2*qi - 2*qf + 2*T*dqf) + 1)*(2*qi - 2*qf + 2*T*dqf)))*((dqf - dqi)/(((dqf*dt - dqi*dt)/(2*qi - 2*qf + 2*T*dqf) - 1) ...
    *(2*qi - 2*qf + 2*T*dqf)) - (dqf - dqi)/(((dqf*dt - dqi*dt)/(2*qi - 2*qf + 2*T*dqf) + 1)*(2*qi - 2*qf + 2*T*dqf))) - ((2^(1/2)*(log((dqf*dt - dqi*dt)/(2*qi - 2*qf + 2*T*dqf) + 1) + log(1 - (dqf*dt - dqi*dt)/(2*qi - 2*qf + 2*T*dqf))))/2 - 1)*((dqf - dqi)^2/(((dqf*dt - dqi*dt)/(2*qi - 2*qf + 2*T*dqf) - 1)^2*(2*qi - 2*qf + 2*T*dqf)^2) - (dqf - dqi)^2/(((dqf*dt - dqi*dt)/(2*qi - 2*qf + 2*T*dqf) + 1)^2*(2*qi - 2*qf + 2*T*dqf)^2)) + (2^(1/2)*(log((dqf*dt - dqi*dt)/(2*qi - 2*qf + 2*T*dqf) + 1) - log(1 - (dqf*dt - dqi*dt)/(2*qi - 2*qf + 2*T*dqf)))*((dqf - dqi)^2/(((dqf*dt - dqi*dt)/(2*qi - 2*qf + 2*T*dqf) - 1)^2*(2*qi - 2*qf + 2*T*dqf)^2) + (dqf - dqi)^2/(((dqf*dt - dqi*dt)/(2*qi - 2*qf + 2*T*dqf) + 1)^2*(2*qi - 2*qf + 2*T*dqf)^2)))/2) + tanh(((2^(1/2)*(log((dqf*dt - dqi*dt)/(2*qi - 2*qf + 2*T*dqf) + 1) + log(1 - (dqf*dt - dqi*dt)/(2*qi - 2*qf + 2*T*dqf))))/2 - 1)*(log((dqf*dt - dqi*dt)/(2*qi - 2*qf + 2*T*dqf) + 1) - log(1 - (dqf*dt - dqi*dt)/(2*qi - 2*qf + 2*T*dqf))))*tanh(log((dqf*dt - dqi*dt)/(2*qi - 2*qf + 2*T*dqf))^2/3 - log(1 - (dqf*dt - dqi*dt)/(2*qi - 2*qf + 2*T*dqf))^2/3)*((2*log((dqf*dt - dqi*dt)/(2*qi - 2*qf + 2*T*dqf))*(dqf - dqi))/(3*(dqf*dt - dqi*dt)) - (2*log(1 - (dqf*dt - dqi*dt)/(2*qi - 2*qf + 2*T*dqf))*(dqf - dqi))/(3*((dqf*dt - dqi*dt)/(2*qi - 2*qf + 2*T*dqf) - 1)*(2*qi - 2*qf + 2*T*dqf)))^2*(tanh(log((dqf*dt - dqi*dt)/(2*qi - 2*qf + 2*T*dqf))^2/3 - log(1 - (dqf*dt - dqi*dt)/(2*qi - 2*qf + 2*T*dqf))^2/3)^2 - 1) - (tanh(((2^(1/2)*(log((dqf*dt - dqi*dt)/(2*qi - 2*qf + 2*T*dqf) + 1) + log(1 - (dqf*dt - dqi*dt)/(2*qi - 2*qf + 2*T*dqf))))/2 - 1)*(log((dqf*dt - dqi*dt)/(2*qi - 2*qf + 2*T*dqf) + 1) - log(1 - (dqf*dt - dqi*dt)/(2*qi - 2*qf + 2*T*dqf))))^2 - 1)*((2*log((dqf*dt - dqi*dt)/(2*qi - 2*qf + 2*T*dqf))*(dqf - dqi))/(3*(dqf*dt - dqi*dt)) - (2*log(1 - (dqf*dt - dqi*dt)/(2*qi - 2*qf + 2*T*dqf))*(dqf - dqi))/(3*((dqf*dt - dqi*dt)/(2*qi - 2*qf + 2*T*dqf) - 1)*(2*qi - 2*qf + 2*T*dqf)))*(tanh(log((dqf*dt - dqi*dt)/(2*qi - 2*qf + 2*T*dqf))^2/3 - log(1 - (dqf*dt - dqi*dt)/(2*qi - 2*qf + 2*T*dqf))^2/3)^2 - 1)*(((2^(1/2)*(log((dqf*dt - dqi*dt)/(2*qi - 2*qf + 2*T*dqf) + 1) + log(1 - (dqf*dt - dqi*dt)/(2*qi - 2*qf + 2*T*dqf))))/2 - 1)*((dqf - dqi)/(((dqf*dt - dqi*dt)/(2*qi - 2*qf + 2*T*dqf) - 1)*(2*qi - 2*qf + 2*T*dqf)) - (dqf - dqi)/(((dqf*dt - dqi*dt)/(2*qi - 2*qf + 2*T*dqf) + 1)*(2*qi - 2*qf + 2*T*dqf))) - (2^(1/2)*(log((dqf*dt - dqi*dt)/(2*qi - 2*qf + 2*T*dqf) + 1) - log(1 - (dqf*dt - dqi*dt)/(2*qi - 2*qf + 2*T*dqf)))*((dqf - dqi)/(((dqf*dt - dqi*dt)/(2*qi - 2*qf + 2*T*dqf) - 1)*(2*qi - 2*qf + 2*T*dqf)) + (dqf - dqi)/(((dqf*dt - dqi*dt)/(2*qi - 2*qf + 2*T*dqf) + 1)*(2*qi - 2*qf + 2*T*dqf))))/2) - tanh(log((dqf*dt - dqi*dt)/(2*qi - 2*qf + 2*T*dqf))^2/3 - log(1 - (dqf*dt - dqi*dt)/(2*qi - 2*qf + 2*T*dqf))^2/3)*((2*log((dqf*dt - dqi*dt)/(2*qi - 2*qf + 2*T*dqf))*(dqf - dqi))/(3*(dqf*dt - ...
    dqi*dt)) - (2*log(1 - (dqf*dt - dqi*dt)/(2*qi - 2*qf + 2*T*dqf))*(dqf - dqi))/(3*((dqf*dt - dqi*dt)/(2*qi - 2*qf + 2*T*dqf) - 1)*(2*qi - 2*qf + 2*T*dqf)))^2*(tanh(log((dqf*dt - dqi*dt)/(2*qi - 2*qf + 2*T*dqf))^2/3 - log(1 - (dqf*dt - dqi*dt)/(2*qi - 2*qf + 2*T*dqf))^2/3)^2 - 1)*(tanh((log(2 - (dqf*dt - dqi*dt)/(2*qi - 2*qf + 2*T*dqf)) - log((dqf*dt - dqi*dt)/(2*qi - 2*qf + 2*T*dqf)))*((2^(1/2)*(log(2 - (dqf*dt - dqi*dt)/(2*qi - 2*qf + 2*T*dqf)) + log((dqf*dt - dqi*dt)/(2*qi - 2*qf + 2*T*dqf))))/2 - 1)) - (2*(dqf*dt - dqi*dt))/(2*qi - 2*qf + 2*T*dqf) + 1) + 2*tanh(((2^(1/2)*(log((dqf*dt - dqi*dt)/(2*qi - 2*qf + 2*T*dqf) + 1) + log(1 - (dqf*dt - dqi*dt)/(2*qi - 2*qf + 2*T*dqf))))/2 - 1)*(log((dqf*dt - dqi*dt)/(2*qi - 2*qf + 2*T*dqf) + 1) - log(1 - (dqf*dt - dqi*dt)/(2*qi - 2*qf + 2*T*dqf))))*(tanh(((2^(1/2)*(log((dqf*dt - dqi*dt)/(2*qi - 2*qf + 2*T*dqf) + 1) + log(1 - (dqf*dt - dqi*dt)/(2*qi - 2*qf + 2*T*dqf))))/2 - 1)*(log((dqf*dt - dqi*dt)/(2*qi - 2*qf + 2*T*dqf) + 1) - log(1 - (dqf*dt - dqi*dt)/(2*qi - 2*qf + 2*T*dqf))))^2 - 1)*(tanh(log((dqf*dt - dqi*dt)/(2*qi - 2*qf + 2*T*dqf))^2/3 - log(1 - (dqf*dt - dqi*dt)/(2*qi - 2*qf + 2*T*dqf))^2/3)/2 - 1/2)*(((2^(1/2)*(log((dqf*dt - dqi*dt)/(2*qi - 2*qf + 2*T*dqf) + 1) + log(1 - (dqf*dt - dqi*dt)/(2*qi - 2*qf + 2*T*dqf))))/2 - 1)*((dqf - dqi)/(((dqf*dt - dqi*dt)/(2*qi - 2*qf + 2*T*dqf) - 1)*(2*qi - 2*qf + 2*T*dqf)) - (dqf - dqi)/(((dqf*dt - dqi*dt)/(2*qi - 2*qf + 2*T*dqf) + 1)*(2*qi - 2*qf + 2*T*dqf))) - (2^(1/2)*(log((dqf*dt - dqi*dt)/(2*qi - 2*qf + 2*T*dqf) + 1) - log(1 - (dqf*dt - dqi*dt)/(2*qi - 2*qf + 2*T*dqf)))*((dqf - dqi)/(((dqf*dt - dqi*dt)/(2*qi - 2*qf + 2*T*dqf) - 1)*(2*qi - 2*qf + 2*T*dqf)) + (dqf - dqi)/(((dqf*dt - dqi*dt)/(2*qi - 2*qf + 2*T*dqf) + 1)*(2*qi - 2*qf + 2*T*dqf))))/2)^2);

qv = [qd;dqd;ddqd]; %Send values back

end

function ris=compute_traj_parameters(s0, v0, sf, vm, am)
    ris=zeros(15,1);
    radix=zeros(2,1);
    T1 = 0;
    dT = 0;
    T2 = 0;
    a1 = 0;
    b1 = 0;
    c1 = 0;
    d1 = 0;
    e1 = 0;
    a2 = 0;
    b2 = 0;
    c2 = 0;
    d2 = 0;
    e2 = 0;
    k = 0;

    if (vm~=0) %check...
        vm=vm*sign(sf-s0);
        k=am*sign(sf-s0);
        T1 = -3/2*(v0-vm)/k;
        a1 = -4/27*k^3/(v0-vm)^2;
        b1 = -4/9*k^2/(v0-vm);
        e1 = s0;
        d1 = v0;
        c1 = 0;
        c2 = 0;
        T2 = 3/2*vm/k;
        dT = 1/4*(-3*vm^2+4*sf*k-4*a1*T1^4*k-4*b1*T1^3*k-4*c1*T1^2*k-4*d1*T1*k-4*e1*k)/vm/k;
        a2 = 4/27*k^3/vm^2;
        d2 = vm;
        e2 = 1/4*(-3*vm^2+4*sf*k)/k;
        b2 = -4/9*k^2/vm;
        if (dT<0)
            c2 = 0;
            c1 = 0;
            a=2;
            b=12*v0;
            c=9*v0^2-12*sf*k+12*s0*k;
            radix(1)=(-b + sqrt(b^2-4*a*c))/(2*a);
            radix(2)=(-b - sqrt(b^2-4*a*c))/(2*a);
            %decide the correct root
            T1_a = 1/2*radix(1)/k;
            T2_a = 1/2*(radix(1)+3*v0)/k;
            T1_b = 1/2*radix(2)/k;
            T2_b = 1/2*(radix(2)+3*v0)/k;
                if (and(T1_a>=0, T2_a>=0))
                    r=radix(1);
                    T1=T1_a;
                    T2=T2_a;
                    dT=0;
                    two_phases=1;
                elseif (and(T1_b>=0, T2_b>=0))
                    r=radix(2);
                    T1=T1_b;
                    T2=T2_b;
                    dT=0;
                    two_phases=1;
                else
                    r=0;
                    two_phases=0;
                end
                if (two_phases==0)
                    T1=0;
                    T2=2*(sf-s0)/v0;
                    dT=0;
                    b2=-1/4*v0^3/(sf-s0)^2;
                    c2=0;
                    a2=1/16*v0^4/(sf-s0)^3;
                    d2=v0;
                    e2=s0;
                else
                    b1 = -8/9*k^2/(4*v0*r+3*v0^2-4*sf*k+4*s0*k)*r;
                    a1 = 8/9*k^3/(4*v0*r+3*v0^2-4*sf*k+4*s0*k);
                    b2 = -8/9*k^2/(4*sf*k+3*v0^2-4*s0*k)*(r+3*v0);
                    e2 = -1/8*(3*v0^2-4*s0*k-4*sf*k)/k;
                    e1 = s0;
                    d1 = v0;
                    d2 = 2/9/(4*sf*k+3*v0^2-4*s0*k)*(r+3*v0)^3;
                    a2 = 8/9*k^3/(4*sf*k+3*v0^2-4*s0*k);
                end
        end
    end
    ris=[T1;dT;T2; a1; b1; c1; d1; e1; a2; b2; c2; d2; e2; vm; k];
end

%time, and the output of the previous function
function [ris, finished]=interpolator(t, parameters)

ris=zeros(3,1);
T1=parameters(1);
dT=parameters(2);
T2=parameters(3);
a1=parameters(4);
b1=parameters(5);
c1=parameters(6);
d1=parameters(7);
e1=parameters(8);
a2=parameters(9);
b2=parameters(10);
c2=parameters(11);
d2=parameters(12);
e2=parameters(13);
vm=parameters(14);
k=parameters(15);

finished = 0;
if (vm~=0) %check...
        if (t<=T1)
            ris=[a1*t^4+b1*t^3+c1*t^2+d1*t+e1; 4*a1*t^3+3*b1*t^2+2*c1*t+d1; 12*a1*t^2+6*b1*t+2*c1];
        elseif (t<=T1+dT)
            t=t-T1;
            ris=[a1*T1^4+b1*T1^3+c1*T1^2+d1*T1+e1+vm*t; vm; 0];
        elseif (t<=T1+dT+T2)
            t=t-T1-dT;
            ris=[a2*t^4+b2*t^3+c2*t^2+d2*t+e2; 4*a2*t^3+3*b2*t^2+2*c2*t+d2; 12*a2*t^2+6*b2*t+2*c2];
        else
            t=T2;
            ris=[a2*t^4+b2*t^3+c2*t^2+d2*t+e2;0;0];
            finished=1;
        end
else
    ris=[0;0;0];
end

end

function t=interpolator_1(q, parameters)

T1=parameters(1);
dT=parameters(2);
T2=parameters(3);
a1=parameters(4);
b1=parameters(5);
c1=parameters(6);
d1=parameters(7);
e1=parameters(8);
a2=parameters(9);
b2=parameters(10);
c2=parameters(11);
d2=parameters(12);
e2=parameters(13);
vm=parameters(14);
k=parameters(15);

t=0;
Q1 = a1*T1^4+b1*T1^3+c1*T1^2+d1*T1+e1;%q point at end of startup
Q2 = a2*T2^4+b2*T2^3+c2*T2^2+d2*T2+e2;%final q
Q3 = Q2-Q1;%q point at end of linear part (using symmetry)

if q<Q1
    %startup
%     %tarray = 0:0.001:T1; %not working, because T1 should be constant?!
%     tarray = linspace(0,T1);
%     qarray=zeros(size(tarray));
%     parfor i=1:size(tarray,2)
%         [qv,~]=interpolator(tarray(i), parameters);
%         qarray(i)=qv(1);
%     end
%     t = interp1(qarray, tarray, q);
    t=0;
    error('trans: interpolator_1 startup: not programmed jet, sry');
    % problem with calculating additional shift
elseif q>=Q1 || q<=Q3
    %linear part
    t = T1+((q-Q1)/vm);
elseif q>Q3
    %slowdown
    t=0;
    error('trans: interpolator_1 slowdown: not programmed jet, sry');
end

end

== matlab function RB_KAIROS_BaseOnly/EE to task space quaternion quantities/Get Pose in quaternions ==
  data: T input; p output; qt output
function [p, qt] = tform2pose_quat(T)
% Retrieves the pose of the end effector using quaternion representation
% for the orientation 

p = T(1:3,4);
qt = tform2quat(T)';

== matlab function RB_KAIROS_BaseOnly/EE to task space quaternion quantities/MATLAB Function ==
  data: qt input; qt_unit output
function qt_unit = qt_norm(qt)

qt_unit = qt./norm(qt);

== matlab function RB_KAIROS_BaseOnly/EE to task space quaternion quantities/MATLAB Function1 ==
  data: R input; qt output
function qt = rotm2quat(R)

qt = rotm2quat(R)';

== matlab function RB_KAIROS_BaseOnly/EE to task space quaternion quantities/MATLAB Function2 ==
  data: qt input; qt_unit output
function qt_unit = qt_norm(qt)

qt_unit = qt./norm(qt);

== matlab function RB_KAIROS_BaseOnly/EE to task space quaternion quantities/MATLAB Function4 ==
  data: qt1 input; qt_prod output; qt2 input
function qt_prod = quat_product(qt1,qt2)
% Computes the halmiton product

% Inverse of desired quaternion

eta1 = qt1(1);
eta2 = qt2(1);

eps1 = qt1(2:4);
eps2 = qt2(2:4);

% Quaternion product qt_EE*qt_des_i
qt_prod = [eta1*eta2-dot(eps1,eps2);
    (eta1*eps2+eta2*eps1+cross(eps1,eps2))];

== matlab function RB_KAIROS_BaseOnly/EE to task space quaternion quantities/Subsystem/S(omega) ==
  data: v input; S output
function S = calc_skewsymm(v)

S = [0 -v(3) v(2);
    v(3) 0 -v(1);
    -v(2) v(1) 0];

== matlab function RB_KAIROS_BaseOnly/EE to task space quaternion quantities/conjugate ==
  data: qt input; qt_i output
function qt_i = quat_conjugate(qt)

qt_i = [qt(1); -qt(2:4)];
